simulink model "SimulacionSistemaControl"  (Simulink 8.9)
settings: Solver=VariableStepAuto  StartTime=0.0  StopTime=10.0  RelTol=1e-3
settings Model: Creator=Helbert  LastModifiedBy=Helbert
settings DataIOCC: LimitDataPoints=off  SaveFormat=Dataset  SignalLoggingSaveFormat=Dataset
settings OptimizationCC: LifeSpan=auto
settings DebuggingCC: UnderspecifiedInitializationDetection=Simplified  MergeDetectMultiDrivingBlocksExec=error  FcnCallInpInsideContextMsg=error  StateNameClashWarn=none  SFUnexpectedBacktrackingDiag=error  SFNoUnconditionalDefaultTransitionDiag=error  SFExecutionAtInitializationDiag=warning
settings HardwareCC: ProdBitPerPointer=64  ProdBitPerSizeT=64  ProdBitPerPtrDiffT=64  ProdLargestAtomicFloat=Float  ProdIntDivRoundTo=Zero  ProdEndianess=LittleEndian  ProdWordSize=64  ProdHWDeviceType=Intel->x86-64 (Windows64)
settings ModelReferenceCC: PropagateSignalLabelsOutOfModel=on
settings GRTTargetCC: TargetLangStandard=C99 (ISO)  GeneratePreprocessorConditionals=Use local settings  CombineOutputUpdateFcns=on  GRTInterface=off
settings ConfigComp: CovMetricSettings=dwe  CovHtmlReporting=off  CovSaveCumulativeToWorkspaceVar=off  CovSaveSingleToWorkspaceVar=off  CovExternalEMLEnable=on

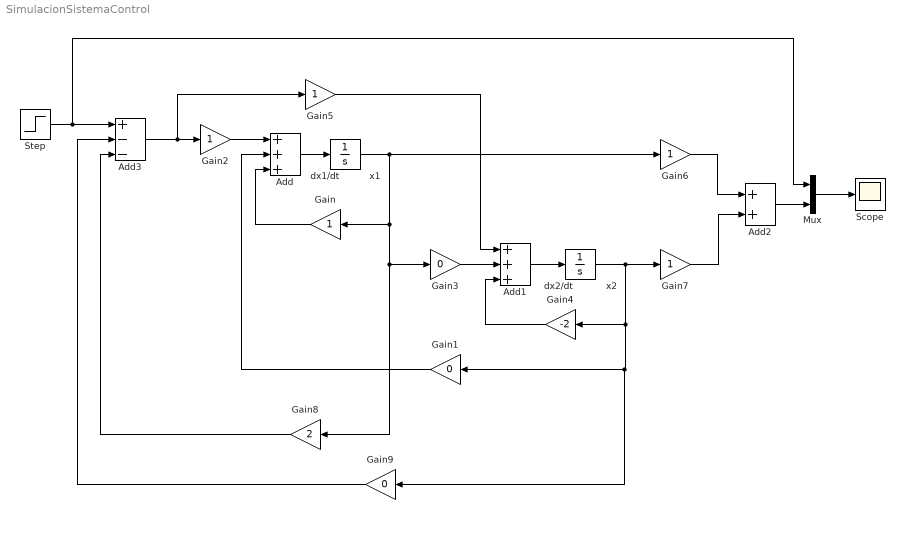
== system SimulacionSistemaControl ==
  Add : Sum  Inputs=+++
  Add1 : Sum  Inputs=+++
  Add2 : Sum
  Add3 : Sum  Inputs=+--
  Gain{,2,5..7} (5 alike) : Gain
  Gain1 : Gain  Gain=0
  Gain3 : Gain  Gain=0
  Gain4 : Gain  Gain=-2
  Gain8 : Gain  Gain=2
  Gain9 : Gain  Gain=0
  Mux : Mux  Inputs=2
  Scope : Scope
  Step : Step  Time=0  SampleTime=0
  dx1/dt          x1 : Integrator
  dx2/dt           x2 : Integrator
  wires:
  Add/1 -> dx1/dt          x1/1
  Add1/1 -> dx2/dt           x2/1
  dx1/dt          x1/1 -> Gain6/1, Gain3/1, Gain8/1, Gain/1
  Gain/1 -> Add/3
  dx2/dt           x2/1 -> Gain7/1, Gain4/1, Gain9/1, Gain1/1
  Gain1/1 -> Add/2
  Gain2/1 -> Add/1
  Gain3/1 -> Add1/2
  Gain4/1 -> Add1/3
  Gain5/1 -> Add1/1
  Gain6/1 -> Add2/1
  Gain7/1 -> Add2/2
  Add3/1 -> Gain5/1, Gain2/1
  Step/1 -> Mux/1, Add3/1
  Gain8/1 -> Add3/3
  Gain9/1 -> Add3/2
  Add2/1 -> Mux/2
  Mux/1 -> Scope/1
